simulink library "Sattelite_PD_Controller"  (R2016a)
settings: Solver=ode45  StartTime=0.0  StopTime=10.0  RelTol=1e-3
undefined symbols (not defined in the file): kd, kp
libraries: Satellite_Dynamics x1
settings Model: Creator=devantormey  LastModifiedBy=devantormey
settings DataIOCC: LimitDataPoints=on
settings DebuggingCC: AllowSymbolicDim=off

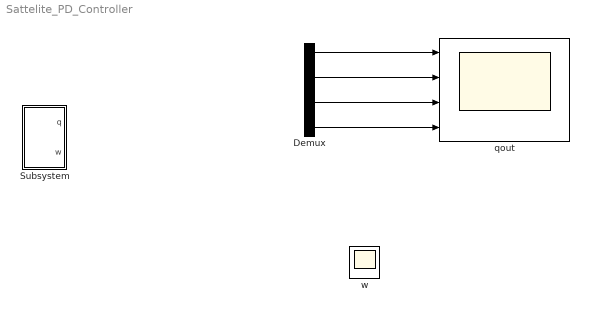
== system Sattelite_PD_Controller ==
  Demux : Demux
  Subsystem : Subsystem
  qout : Scope  NumInputPorts=4
  w : Scope
  wires:
  Demux/1 -> qout/1
  Demux/2 -> qout/2
  Demux/3 -> qout/3
  Demux/4 -> qout/4

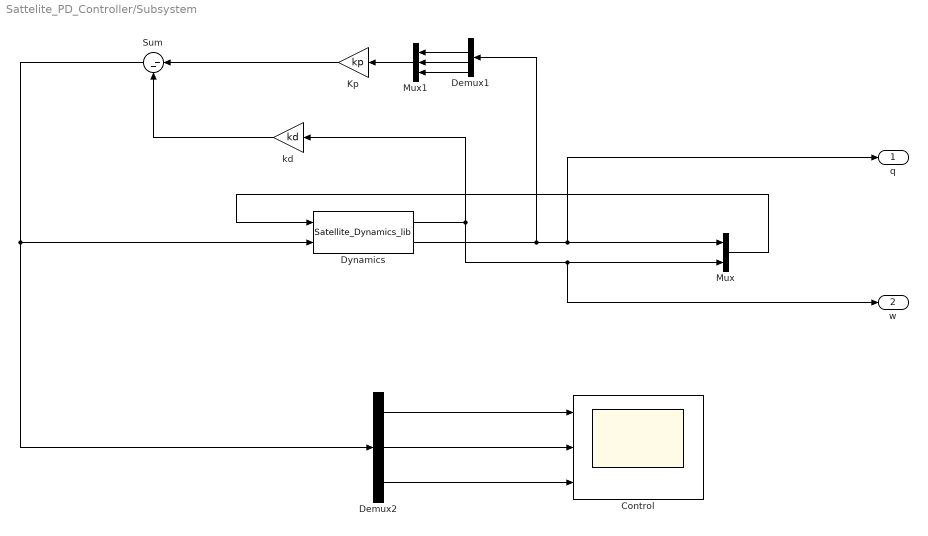
== system Sattelite_PD_Controller/Subsystem ==
  Control : Scope  NumInputPorts=3
  Demux1 : Demux
  Demux2 : Demux  Outputs=3
  "Dynamics " : Satellite_Dynamics/Satellite_Dynamics_lib
  Kp : Gain  Gain=kp
  Mux : Mux  Inputs=2
  Mux1 : Mux  Inputs=3
  Sum : Sum  Inputs=|--
  kd : Gain  Gain=kd
  q : Outport
  w : Outport  Port=2
  wires:
  "Dynamics "/2 -> Demux1/1, q/1, Mux/1
  Mux/1 -> "Dynamics "/1
  "Dynamics "/1 -> kd/1, w/1, Mux/2
  kd/1 -> Sum/2
  Sum/1 -> "Dynamics "/2, Demux2/1
  Mux1/1 -> Kp/1
  Demux1/2 -> Mux1/1
  Demux1/3 -> Mux1/2
  Demux1/4 -> Mux1/3
  Demux2/2 -> Control/2
  Demux2/1 -> Control/1
  Demux2/3 -> Control/3
  Kp/1 -> Sum/1
